simulink model "Gimbal_Control"  (R2025b)
settings: Solver=FixedStepAuto  StartTime=0.0  StopTime=10.0  FixedStep=0.001  RelTol=1e-3
libraries: simulink_extras x2
settings Model: Creator=user  LastModifiedBy=lew11

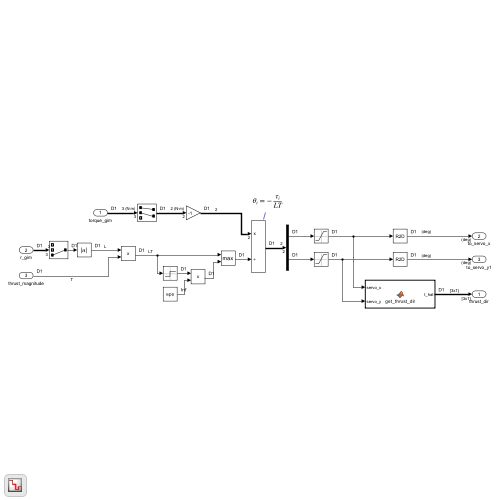
[thumbnail: Simulink's stored preview of the top-level diagram]
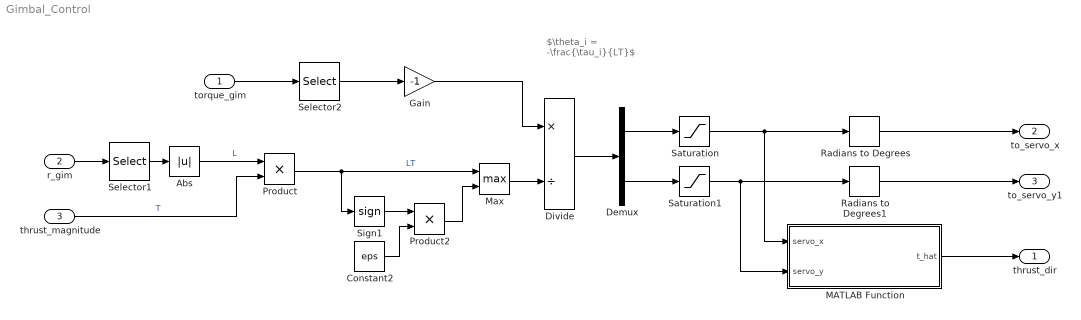
== system Gimbal_Control ==
  note: $\theta_i = -\frac{\tau_i}{LT}$
  torque_gim : Inport  Unit=N*m  PortDimensions=3
  r_gim : Inport  Port=2  PortDimensions=3
  thrust_magnitude : Inport  Port=3  PortDimensions=1
  Abs : Abs  SaturateOnIntegerOverflow=off
  Constant2 : Constant  Value=eps
  Demux : Demux  Outputs=2
  Divide : Product  Inputs=*/
  Gain : Gain  Gain=-1
  MATLAB Function : MATLAB Function  TreatAsAtomicUnit=on
  Max : MinMax  Function=max  Inputs=2
  Product : Product
  Product2 : Product
  Radians to Degrees : simulink_extras/Transformations/Radians to Degrees
  Radians to Degrees1 : simulink_extras/Transformations/Radians to Degrees
  Saturation : Saturate  UpperLimit=deg2rad(15)  LowerLimit=deg2rad(-15)
  Saturation1 : Saturate  UpperLimit=deg2rad(15)  LowerLimit=deg2rad(-15)
  Selector1 : Selector  InputPortWidth=3  IndexOptions=Index vector (dialog)  Indices=[3]  OutputSizes=1
  Selector2 : Selector  InputPortWidth=3  IndexOptions=Index vector (dialog)  Indices=[1 2]  OutputSizes=1
  Sign1 : Signum
  thrust_dir : Outport
  to_servo_x : Outport  Port=2  Unit=deg  PortDimensions=1
  to_servo_y1 : Outport  Port=3  Unit=deg  PortDimensions=1
  wires:
  Demux/1 -> Saturation/1
  Gain/1 -> Divide/1
  thrust_magnitude/1 -> Product/2  "T"
  Saturation1/1 -> MATLAB Function/2(servo_y), Radians to Degrees1/1
  r_gim/1 -> Selector1/1
  Selector2/1 -> Gain/1
  Divide/1 -> Demux/1
  Max/1 -> Divide/2
  torque_gim/1 -> Selector2/1
  Demux/2 -> Saturation1/1
  Saturation/1 -> MATLAB Function/1(servo_x), Radians to Degrees/1
  Abs/1 -> Product/1  "L"
  MATLAB Function/1(t_hat) -> thrust_dir/1
  Selector1/1 -> Abs/1
  Product2/1 -> Max/2
  Constant2/1 -> Product2/2
  Sign1/1 -> Product2/1
  Product/1 -> Sign1/1, Max/1  "LT"
  Radians to Degrees/1 -> to_servo_x/1
  Radians to Degrees1/1 -> to_servo_y1/1

== matlab function Gimbal_Control/MATLAB Function ==
  data: servo_x input; t_hat output; servo_y input
function t_hat = get_thrust_dir(servo_x, servo_y)

t_x = -servo_y;
t_y = servo_x;
t_z = -1 + (servo_x^2+servo_y^2)/2;

t_hat = [t_x; t_y; t_z];
